simulink model "dspldm"  (Simulink 4.00)
settings: Solver=ode5  SolverMode=SingleTasking  StartTime=0.0  StopTime=99999  FixedStep=1/64000  MaxStep=1/64000  RelTol=1e-3  AbsTol=1e-6
libraries: dspwvfmcdlib x2, dspddes2 x1, simulink3 x1
settings Model: Creator=don  LastModifiedBy=asharma  SaveTime=off  SaveOutput=off  LimitDataPoints=off  IntegerOverflowMsg=none  ExtModeTrigMode=oneshot  ExtModeArmWhenConnect=off  BlockReductionOpt=off

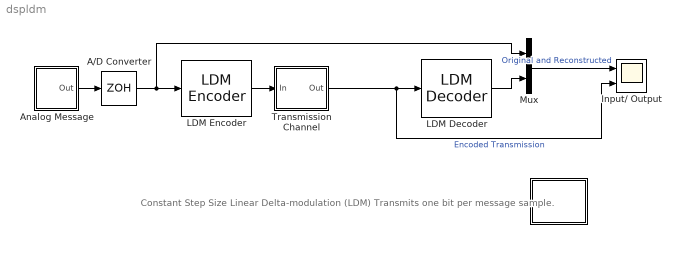
== system dspldm ==
  note: Constant Step Size
      | Linear Delta-modulation (LDM)
      |
      | Transmits one bit per message sample.
  " " : Subsystem
      settings: RTWFcnNameOpts=Auto  RTWFileNameOpts=Auto
      mask Type: LDM Info block
      mask Display: disp('Info')
  A/D Converter : ZeroOrderHold  SampleTime=1/8000
  Analog Message : Subsystem
      settings: RTWFcnNameOpts=Auto  RTWFileNameOpts=Auto
  Input/ Output : Scope  NumInputPorts=2
      settings: TimeRange=0.02  YMin=-1.5~-0.1  YMax=1.5~1.1  SaveToWorkspace=off  SaveName=ScopeData  DataFormat=Array  LimitDataPoints=on  MaxDataPoints=5000
  LDM Decoder : dspwvfmcdlib/LDM Decoder  Tau=0.91
  LDM Encoder : dspwvfmcdlib/LDM Encoder  EncTau=0.91
  Mux : Mux  Inputs=2
  Transmission Channel : Subsystem
      settings: RTWFcnNameOpts=Auto  RTWFileNameOpts=Auto
  wires:
  Mux/1 -> Input/ Output/1  "Original and Reconstructed"
  Transmission Channel/1(Out) -> LDM Decoder/1, Input/ Output/2  "Encoded Transmission"
  A/D Converter/1 -> Mux/1, LDM Encoder/1
  Analog Message/1(Out) -> A/D Converter/1
  LDM Decoder/1 -> Mux/2
  LDM Encoder/1 -> Transmission Channel/1(In)

== system dspldm/  ==
  note: Linear Delta-modulation (LDM)  is a modification of Delta-Modulation (DM).
      |
      | Delta Modulation (DM) is a differential waveform quantization (or coding) technique. A DM
      | encoder uses the error between the original signal to be coded and the coded signal itself
      | to create a differentially-quantized data stream. This data stream (usually the computed error
      | signal) is a lower bit-rate signal that can be decoded  by a matched decoder on the receiver
      | side in order to achieve data compression and hence low data transmission rates.
      |
      | LDM employs two-level (i.e. one-bit) encoders, and may be performed at many different
      | sampling/data rates. The encoded bit rate is usually directly proportional to the input signal
      | sample rate. In LDM, a constant step-size is used to approximate the input signal with a
      | single-bit per signal sample. In the encoded bit-stream, each "1" bit means "increase the
      | amplitude" by the step-size (as compared to the previous decoded signal sample), while a
      | "0" bit means "decrease the amplitude" by the step-size (as compared to the previous
      | decoded signal sample). Using LDM, the encoder performance can suffer due to a condition
      | known as "slope overload", then the input signal slope (such as during high frequency
      | content) changes too rapidly for the encoder to track it accurately.

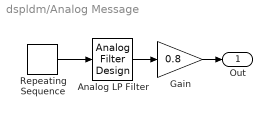
== system dspldm/Analog Message ==
  Analog LP Filter : dspddes2/Analog Filter Design  method=Butterworth  filttype=Lowpass  N=5  Wlo=2*pi*400  Whi=80  Rp=3  Rs=40
  Gain : Gain  Gain=0.8  Multiplication=Element-wise(K.*u)  SaturateOnIntegerOverflow=on
  Repeating Sequence : simulink3/Sources/Repeating Sequence  rep_seq_t=[0 .005 .005 .015 .015 .02]  rep_seq_y=[1 1 -1 -1 1 1]
  Out : Outport  Port=1  InitialOutput=0
  wires:
  Analog LP Filter/1 -> Gain/1
  Repeating Sequence/1 -> Analog LP Filter/1
  Gain/1 -> Out/1

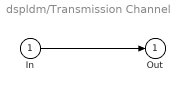
== system dspldm/Transmission Channel ==
  In : Inport  Port=1
  Out : Outport  Port=1  InitialOutput=0
  wires:
  In/1 -> Out/1
